simulink model "JX_Kinect3"  (Simulink 7.7)
settings: Solver=ode4  StartTime=0.0  StopTime=inf  FixedStep=sample_time  RelTol=1e-3
InitFcn:
  | sample_time=0.005;%0.004;%0.0025;%0.02;
  | DeltaT = 0.02;
  | g = 9.81;
  | H0 = g%0.3165;
  | Kl = 1;
  | 
  | Omega_r = 1.6;%for Horizontal reference
  | Zeta_r = 1; %for Horizontal reference
  | Omega = 1.8;%for Horizontal Control
  | Zeta = 0.5;    %for Horizontal Control
  | 
  | Omega_h_r = 2.5; %for vertical reference
  | Zeta_h_r = 0.8;  %for vertical reference
  | Omega_h = 2.7;    %for vertical control
  | Zeta_h = 0.8;         %for vertical control
  | PI=pi;
  | 
  | Mass = 1.15;
  | Acc_Max = 4;
  | Acc_Max_h = 4;
  | 
  | Max_RP = 60;
  | 
  | % for NN
  | n = 5;
  | r = 3;
  | n2 = 5;
  | NN_ST = 0.02;
  | 
  | GAMA_V = 6;
  | gama_V_e = 0.01;
  | 
  | GAMA_W = GAMA_V;
  | gama_W_e =0.01;
  | 
  | % deadzone
  | NN_Deadzone_Z = 0;
  | 
  | % inputs nomalizaton parameters
  | NN_Z_y_min = -3;
  | NN_Z_y_max = 0.5;
  | 
  | NN_Z_v_max = 8;
  | NN_Z_v_min = -NN_Z_v_max;
  | 
  | % alpha = 0.034;
  | alpha = 1;
  | % c_f = 0.0015;
  | c_f = 0.001;
  | c_y_tilt = 1*0.5;
  | 
  | %for WK paras
  | Heightcontrol = 0.08;
  | Scale_Factor=1;
  | yoffset=0;
  | 
  | load MaoBi_Oct04_2_int.mat
  | MB_Interp.time = [];
undefined symbols (not defined in the file or in its folder): DiscIntNeverNeededParam
libraries: simulink x7, dspadpt3 x3, nid_lib x2, X330_Control x2
(part 3 of 3)

== stateflow chart Planning/Trajectory Logic/UAV SF ==
  state Landing
    state Descending
      en:PosDesired = Pos;
      du:PosDesired[2] = (0.1- PosDesired[2])*1*DeltaT + PosDesired[2] ;
    state CutThrottle
      en: PWM=1600;
      du:HoverThrottle = (0.0- HoverThrottle)*3*DeltaT + HoverThrottle ;
    (default) -> Descending
    Descending -> CutThrottle : [Pos[2] >(0.0 -0.1)]
  state AirBorne
    state TakeOff
      du:HoverThrottle = (H0 - HoverThrottle)*3*DeltaT + HoverThrottle ;
    state Kinect
      state Initialise
        en:
        PosDesired[0]=0, PosDesired[1]=-0,PosDesired[2]= -1.5,PosDesired[3]=0;
        LeftRight = 0;
        UpDown = 0;
        FrontBack = 0;
        ClawStatus = 1;
        Rotation = 0;
        PWM = 1695;
      state Hover
        en:
        PosDesired[0]=0+LeftRight, PosDesired[1]=0+FrontBack,PosDesired[2]= -1.5+UpDown,PosDesired[3] = 0+Rotation;
        LHRH = 0;
        XYZchecker=0;
      state KinectTrack
        state CheckLEFTY
          state YCenter
            en:
            FrontBack=FrontBack+0;
            LHRH = 2;
          state YFront
            en:
            FrontBack=FrontBack-0.02;
            LHRH = 2;
          state YBack
            en:
            FrontBack=FrontBack+0.02;
            LHRH = 2;
          (default) -> (junction 56)
          (junction 56) -> YFront [order 3] : [LeftHand[3]==1]
          (junction 56) -> YCenter [order 2] : [LeftHand[4]==1]
          (junction 56) -> YBack [order 1] : [LeftHand[5]==1]
        state CheckLEFTZ
          state ZCenter
            en:
            UpDown=UpDown+0;
            LHRH = 3;
          state ZDown
            en:
            UpDown=UpDown+0.02;
            LHRH = 3;
          state ZUp
            en:
            UpDown=UpDown-0.02;
            LHRH = 3;
          (junction 57) -> ZUp [order 3] : [LeftHand[6]==1]
          (junction 57) -> ZDown [order 1] : [LeftHand[8]==1]
          (junction 57) -> ZCenter [order 2] : [LeftHand[7]==1]
          (default) -> (junction 57)
        state CheckLEFTX
          state XLeft
            en:
            LeftRight=LeftRight-0.02;
            LHRH=1;
          state XRight
            en:
            LeftRight=LeftRight+0.02;
            LHRH=1;
          state XCenter
            en:
            LeftRight=LeftRight+0;
            LHRH=1;
          (junction 55) -> XRight [order 1] : [LeftHand[2]==1]
          (default) -> (junction 55)
          (junction 55) -> XLeft [order 3] : [LeftHand[0]==1]
          (junction 55) -> XCenter [order 2] : [LeftHand[1]==1]
        state CheckRIGHTXY
          state Anticlockwise
            en:
            Rotation=Rotation+0.2;
            LHRH=4;
          state Neutral
            en:
            Rotation = Rotation +0;
            LHRH = 4;
          state Clockwise
            en:
            Rotation = Rotation - 0.2;
            LHRH = 4;
          state RightHanddown
            en:
            LHRH = 4;
          state CLAW
            state OpenMax
              en:
              PWM = 1695;
              ClawStatus = 0;
              LHRH = 4;
            state CloseMax
              en:
              PWM = 1200;
              ClawStatus = 1;
              LHRH = 4;
            state OpenClaw
              en:
              PWM = PWM+100;
              LHRH = 4;
            state CloseClaw
              en:
              PWM = PWM-100;
              LHRH = 4;
            (junction 67) -> (junction 64) [order 1] : [ClawStatus==0]
            (junction 67) -> (junction 66) [order 2] : [ClawStatus==1]
            (junction 66) -> OpenMax [order 1] : [PWM==1695]
            (junction 66) -> OpenClaw [order 2] : [PWM~=1695]
            (junction 64) -> CloseClaw [order 2] : [PWM~=1200]
            (junction 64) -> CloseMax [order 1] : [PWM==1200]
            (default) -> (junction 67)
          (default) -> (junction 63)
          (junction 63) -> CLAW [order 3] : [RightHand[3]==1]
          (junction 65) -> Anticlockwise [order 3] : [RightHand[0]==1]
          (junction 65) -> Clockwise [order 1] : [RightHand[2]==1]
          (junction 65) -> Neutral [order 2] : [RightHand[1]==1]
          (junction 63) -> RightHanddown [order 2] : [RightHand[5]==1]
          (junction 63) -> (junction 65) [order 1] : [RightHand[4]==1]
        state Finishcycle
          en:
          LHRH = 5;
        CheckLEFTX -> CheckLEFTY : [(LHRH==1)]
        CheckLEFTY -> CheckLEFTZ : [(LHRH==2)]
        (junction 61) -> CheckLEFTX [order 2] : [LeftHand[8]~=2]
        CheckLEFTZ -> CheckRIGHTXY : [(LZcounter==3)]
        (default) -> (junction 61)
        (junction 61) -> (junction 62) [order 1] : [LeftHand[8]==2]
        (junction 62) -> CheckRIGHTXY [order 2] : [RightHand[5]==0]
        (junction 62) -> Finishcycle [order 1] : [RightHand[5]==1]
        CheckRIGHTXY -> Finishcycle : [LHRH ==4]
      state PositionConstraint
        state Xpositive
          en:
          LeftRight=2;
          XYZchecker =1;
        state Xnegative
          en:
          LeftRight=-2;
          XYZchecker=1;
        state Ypositive
          en:
          FrontBack=2;
          XYZchecker=1;
        state Ynegative
          en:
          FrontBack=-2;
          XYZchecker=1;
        state Zpositive
          en:
          FrontBack=1;
          XYZchecker=1;
        state Znegative
          en:
          FrontBack=-1.5;
          XYZchecker=1;
        (junction 60) -> Znegative [order 3] : [UpDown<-1.5]
        (default) -> (junction 60)
        (junction 60) -> Xpositive [order 6] : [LeftRight>2]
        (junction 60) -> Xnegative [order 1] : [LeftRight<-2]
        (junction 60) -> Ypositive [order 5] : [FrontBack>2]
        (junction 60) -> Ynegative [order 2] : [FrontBack<-2]
        (junction 60) -> Zpositive [order 4] : [UpDown>1]
      state ResetChecker
        en:
        XYZchecker=0;
      Hover -> (junction 58) : after (0.02,sec)
      KinectTrack -> Hover [order 2] : [KinectTracking==0]
      (junction 58) -> KinectTrack : [KinectTracking==1]
      KinectTrack -> (junction 59) [order 1] : [(LHRH==5)]
      (default) -> Initialise
      Initialise -> Hover : after (3,sec)
      (junction 59) -> PositionConstraint [order 2] : [(LeftRight > 2)|(LeftRight<-2)|(FrontBack>2)|(FrontBack<-2)|(UpDown>1) | (UpDown<-1.5)]
      (junction 59) -> Hover [order 1] : [(LeftRight<=2)&(LeftRight>=-2)&(FrontBack<=2)&(FrontBack>=-2)&(UpDown<=1)&(UpDown>=-1.5)]
      PositionConstraint -> ResetChecker : [XYZchecker==1]
      ResetChecker -> (junction 59)
    state Safety
      state Descent1
        descentrate=descentrate+0.02;
      state Descent
        en:PosDesired[0] = PerchPos[0]; PosDesired[1] = PerchPos[1];PosDesired[2] = PerchPos[2]-0.50+descentrate;
      state Prelanding
        en:PosDesired[0] = PerchPos[0]; PosDesired[1] = PerchPos[1];PosDesired[2] = PerchPos[2]-0.8 ;
        descentrate=0;
      state SafyHover
        en:PosDesired = Pos; PosDesired[2]= -1.5;
      (default) -> SafyHover
      Descent1 -> Descent : after (0.5,sec)
      Descent -> Descent1 [order 2] : [PerchError < 0.02]
      Descent -> Prelanding [order 1] : after (5,sec)
      Prelanding -> Descent : [PerchError < 0.01]
      SafyHover -> Prelanding : after (3, sec)
    (default) -> TakeOff : {PosDesired = Pos;  PosDesired[2] =-1.2;}
    TakeOff -> Kinect [order 1] : after (7,sec)
    TakeOff -> Safety [order 2] : [RC[5] > 0.5]
    Kinect -> Safety : [RC[5] > 0.5]
  (default) -> Landing : {HoverThrottle = 0;}
  AirBorne -> Landing : [RC[6] < -0.5]
  Landing -> AirBorne : [RC[6] > 0.5]
  data: PosDesired output double size=4; HoverThrottle output double size=1; Mode output uint8 size=1; RC input double size=8; Pos input double size=4; PerchPos input double size=4; DeltaT parameter double size=1; H0 parameter double size=1; Kl parameter double size=1; VelCmd local double size=2 =0; PWM output double; PerchError input double; PI parameter double size=1; draw input double size=3; descentrate local double; LeftHand input double; KinectTracking input double; UpDown local double; FrontBack local double; XYZchecker local double; RightHand input double; ClawStatus local double; LHRH local double; Rotation local double; LeftRight local double
